simulink model "TempCorrect_OfflineTest"  (R2014a)
settings: Solver=ode3  StartTime=0.0  StopTime=1130  FixedStep=1/400  RelTol=1e-3
settings Model: ExtModeTrigDuration=40001  Creator=darenlee  LastModifiedBy=darenlee
settings DataIOCC: SignalLoggingSaveFormat=ModelDataLogs
settings DebuggingCC: MultiTaskDSMMsg=warning  MultiTaskCondExecSysMsg=none
settings RTWCC: IncludeERTFirstTime=on

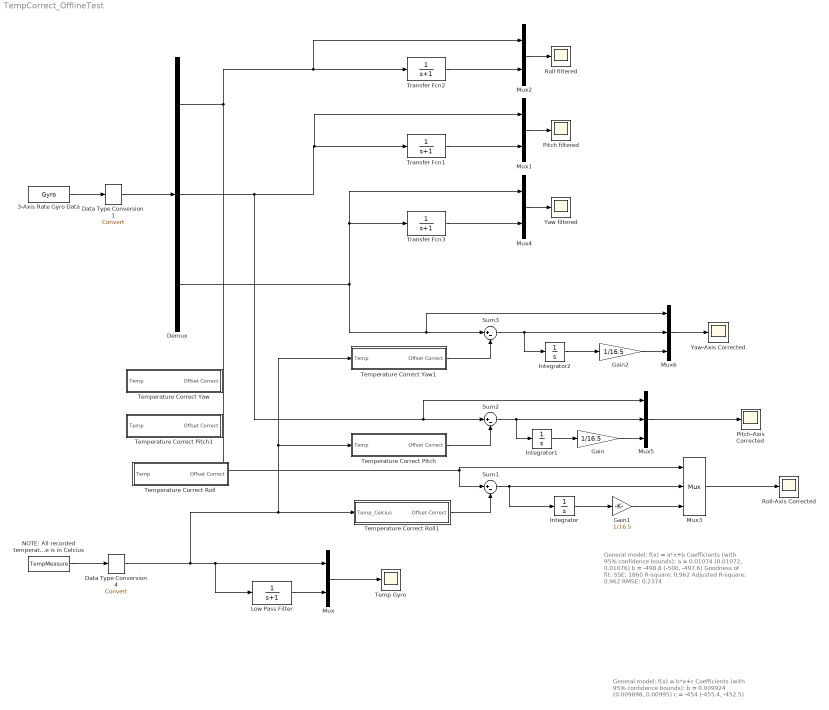
== system TempCorrect_OfflineTest ==
  note: General model:
      |      f(x) = b*x+c
      | Coefficients (with 95% confidence bounds):
      |        b =    0.009924  (0.009898, 0.00995)
      |        c =        -454  (-455.4, -452.5)
  note: General model:
      |      f(x) = a*x+b
      | Coefficients (with 95% confidence bounds):
      |        a =     0.01074  (0.01072, 0.01076)
      |        b =      -498.8  (-500, -497.6)
      |
      | Goodness of fit:
      |   SSE: 1860
      |   R-square: 0.962
      |   Adjusted R-square: 0.962
      |   RMSE: 0.2374
  3-Axis Rate Gyro Data : FromWorkspace  VariableName=Gyro
  Data Type Conversion1 : DataTypeConversion
  Data Type Conversion4 : DataTypeConversion
  Demux : Demux  Outputs=3
  Gain : Gain  Gain=1/16.5
  Gain1 : Gain  Gain=1/16.5
  Gain2 : Gain  Gain=1/16.5
  Integrator : Integrator
  Integrator1 : Integrator
  Integrator2 : Integrator
  Low Pass Filter : TransferFcn  Denominator=[1 1]
  Mux{,1..2,4} (4 alike) : Mux  Inputs=2
  Mux3 : Mux  Inputs=3
  Mux5 : Mux  Inputs=3
  Mux6 : Mux  Inputs=3
  NOTE: All recorded temperature is in Celcius : FromWorkspace  VariableName=TempMeasure
  Pitch filtered : Scope
      settings: SaveName=Pitch_Gyro_filtered
  Pitch-Axis Corrected : Scope
      settings: YMin=-50  YMax=1000  SaveName=Pitch_Corrected_Uncorrected
  Roll filtered : Scope
      settings: SaveName=Roll_Gyro_filtered
  Roll-Axis Corrected : Scope
      settings: TimeRange=571.1351351351351  YMin=-100  YMax=600  SaveName=Roll_Corrected_Uncorrected
  Sum1 : Sum  Inputs=|+-
  Sum2 : Sum  Inputs=|+-
  Sum3 : Sum  Inputs=|+-
  Temp Gyro : Scope
      settings: YMin=0  YMax=55000  SaveName=FilteredTemp
  Temperature Correct Pitch : Subsystem
  Temperature Correct Pitch1 : Subsystem
  Temperature Correct Roll : Subsystem
  Temperature Correct Roll1 : Subsystem
  Temperature Correct Yaw : Subsystem
  Temperature Correct Yaw1 : Subsystem
  Transfer Fcn1 : TransferFcn  Denominator=[1 1]
  Transfer Fcn2 : TransferFcn  Denominator=[1 1]
  Transfer Fcn3 : TransferFcn  Denominator=[1 1]
  Yaw filtered : Scope
      settings: SaveName=Yaw_Gyro_filtered
  Yaw-Axis Corrected : Scope
      settings: YMin=0  YMax=3000  SaveName=Roll_Corrected_Uncorrected2
  wires:
  3-Axis Rate Gyro Data/1 -> Data Type Conversion1/1
  NOTE: All recorded temperature is in Celcius/1 -> Data Type Conversion4/1
  Data Type Conversion1/1 -> Demux/1
  Demux/1 -> Sum1/1, Mux3/1, Mux2/1, Transfer Fcn2/1
  Data Type Conversion4/1 -> Temperature Correct Roll1/1(Temp_Celcius), Temperature Correct Yaw1/1(Temp), Temperature Correct Pitch/1(Temp), Mux/1, Low Pass Filter/1
  Mux/1 -> Temp Gyro/1
  Transfer Fcn2/1 -> Mux2/2
  Sum1/1 -> Integrator/1, Mux3/2
  Mux3/1 -> Roll-Axis Corrected/1
  Mux2/1 -> Roll filtered/1
  Transfer Fcn1/1 -> Mux1/2
  Mux1/1 -> Pitch filtered/1
  Demux/3 -> Mux6/1, Sum3/1, Mux4/1, Transfer Fcn3/1
  Transfer Fcn3/1 -> Mux4/2
  Mux4/1 -> Yaw filtered/1
  Mux5/1 -> Pitch-Axis Corrected/1
  Sum2/1 -> Integrator1/1, Mux5/2
  Low Pass Filter/1 -> Mux/2
  Demux/2 -> Mux5/1, Sum2/1, Mux1/1, Transfer Fcn1/1
  Temperature Correct Pitch/1(Offset Correct) -> Sum2/2
  Temperature Correct Roll1/1(Offset Correct) -> Sum1/2
  Mux6/1 -> Yaw-Axis Corrected/1
  Sum3/1 -> Integrator2/1, Mux6/2
  Temperature Correct Yaw1/1(Offset Correct) -> Sum3/2
  Integrator/1 -> Gain1/1
  Integrator1/1 -> Gain/1
  Gain/1 -> Mux5/3
  Gain1/1 -> Mux3/3
  Integrator2/1 -> Gain2/1
  Gain2/1 -> Mux6/3

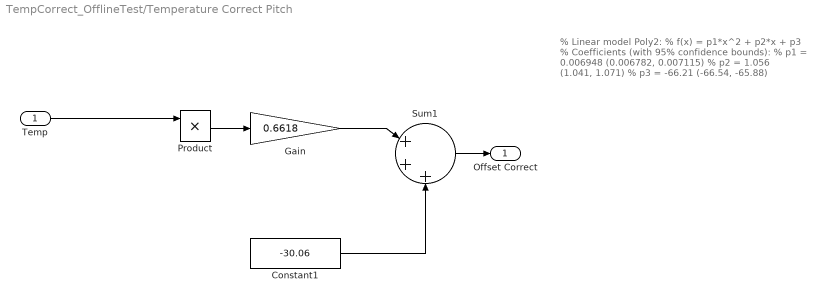
== system TempCorrect_OfflineTest/Temperature Correct Pitch ==
  note: % Linear model Poly2:
      | %      f(x) = p1*x^2 + p2*x + p3
      | % Coefficients (with 95% confidence bounds):
      | %        p1 =    0.006948  (0.006782, 0.007115)
      | %        p2 =       1.056  (1.041, 1.071)
      | %        p3 =      -66.21  (-66.54, -65.88)
  Temp : Inport
  Constant1 : Constant  Value=-30.06
  Gain : Gain  Gain=0.6618
  Product : Product
  Sum1 : Sum  Inputs=|+++
  Offset Correct : Outport
  wires:
  Temp/1 -> Product/1
  Product/1 -> Gain/1
  Gain/1 -> Sum1/1
  Constant1/1 -> Sum1/3
  Sum1/1 -> Offset Correct/1

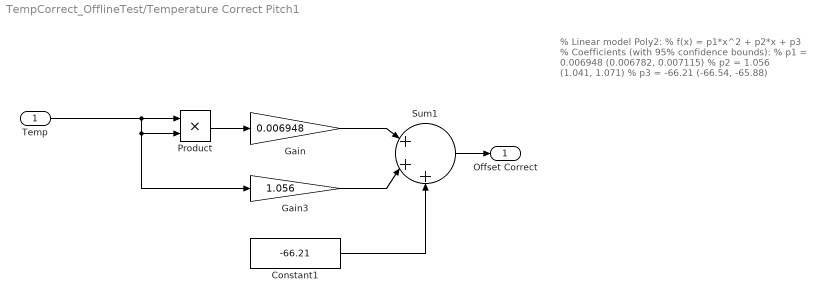
== system TempCorrect_OfflineTest/Temperature Correct Pitch1 ==
  note: % Linear model Poly2:
      | %      f(x) = p1*x^2 + p2*x + p3
      | % Coefficients (with 95% confidence bounds):
      | %        p1 =    0.006948  (0.006782, 0.007115)
      | %        p2 =       1.056  (1.041, 1.071)
      | %        p3 =      -66.21  (-66.54, -65.88)
  Temp : Inport
  Constant1 : Constant  Value=-66.21
  Gain : Gain  Gain=0.006948
  Gain3 : Gain  Gain=1.056
  Product : Product
  Sum1 : Sum  Inputs=|+++
  Offset Correct : Outport
  wires:
  Temp/1 -> Product/1, Gain3/1, Product/2
  Product/1 -> Gain/1
  Gain/1 -> Sum1/1
  Gain3/1 -> Sum1/2
  Constant1/1 -> Sum1/3
  Sum1/1 -> Offset Correct/1

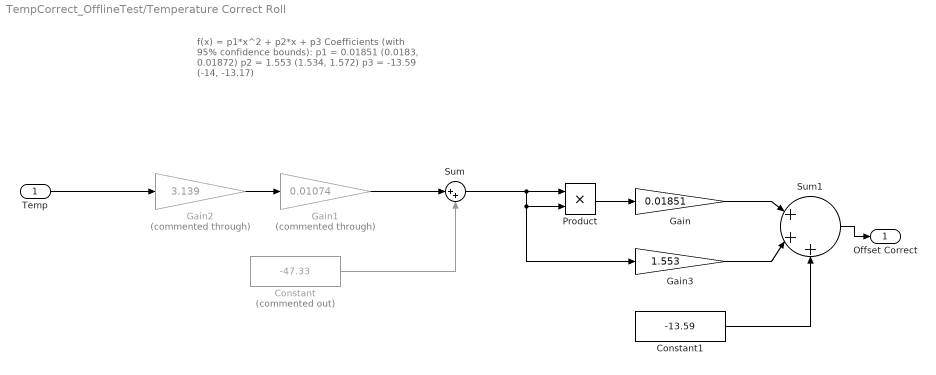
== system TempCorrect_OfflineTest/Temperature Correct Roll ==
  note: f(x) = p1*x^2 + p2*x + p3
      | Coefficients (with 95% confidence bounds):
      |        p1 =     0.01851  (0.0183, 0.01872)
      |        p2 =       1.553  (1.534, 1.572)
      |        p3 =      -13.59  (-14, -13.17)
  Temp : Inport
  Constant : Constant  Commented=on  Value=-47.33
  Constant1 : Constant  Value=-13.59
  Gain : Gain  Gain=0.01851
  Gain1 : Gain  Commented=through  Gain=0.01074
  Gain2 : Gain  Commented=through  Gain=3.139
  Gain3 : Gain  Gain=1.553
  Product : Product
  Sum : Sum  Inputs=|++
  Sum1 : Sum  Inputs=|+++
  Offset Correct : Outport
  wires:
  Gain2/1 -> Gain1/1
  Constant/1 -> Sum/2
  Sum/1 -> Product/1, Gain3/1, Product/2
  Gain1/1 -> Sum/1
  Temp/1 -> Gain2/1
  Product/1 -> Gain/1
  Gain/1 -> Sum1/1
  Gain3/1 -> Sum1/2
  Constant1/1 -> Sum1/3
  Sum1/1 -> Offset Correct/1

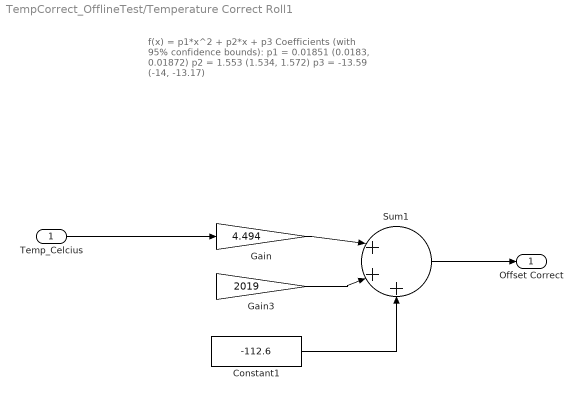
== system TempCorrect_OfflineTest/Temperature Correct Roll1 ==
  note: f(x) = p1*x^2 + p2*x + p3
      | Coefficients (with 95% confidence bounds):
      |        p1 =     0.01851  (0.0183, 0.01872)
      |        p2 =       1.553  (1.534, 1.572)
      |        p3 =      -13.59  (-14, -13.17)
  Temp_Celcius : Inport
  Constant1 : Constant  Value=-112.6
  Gain : Gain  Gain=4.494
  Gain3 : Gain  Gain=2019
  Sum1 : Sum  Inputs=|+++
  Offset Correct : Outport
  wires:
  Temp_Celcius/1 -> Gain/1
  Gain/1 -> Sum1/1
  Gain3/1 -> Sum1/2
  Constant1/1 -> Sum1/3
  Sum1/1 -> Offset Correct/1

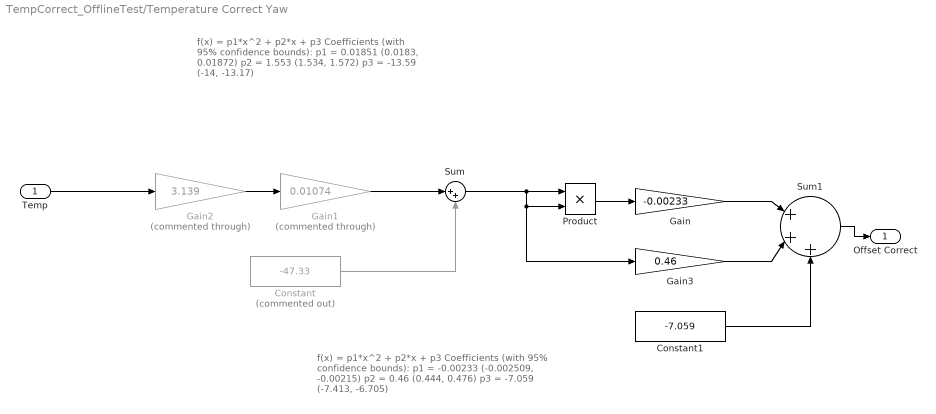
== system TempCorrect_OfflineTest/Temperature Correct Yaw ==
  note: f(x) = p1*x^2 + p2*x + p3
      | Coefficients (with 95% confidence bounds):
      |        p1 =     0.01851  (0.0183, 0.01872)
      |        p2 =       1.553  (1.534, 1.572)
      |        p3 =      -13.59  (-14, -13.17)
  note: f(x) = p1*x^2 + p2*x + p3
      | Coefficients (with 95% confidence bounds):
      |        p1 =    -0.00233  (-0.002509, -0.00215)
      |        p2 =        0.46  (0.444, 0.476)
      |        p3 =      -7.059  (-7.413, -6.705)
  Temp : Inport
  Constant : Constant  Commented=on  Value=-47.33
  Constant1 : Constant  Value=-7.059
  Gain : Gain  Gain=-0.00233
  Gain1 : Gain  Commented=through  Gain=0.01074
  Gain2 : Gain  Commented=through  Gain=3.139
  Gain3 : Gain  Gain=0.46
  Product : Product
  Sum : Sum  Inputs=|++
  Sum1 : Sum  Inputs=|+++
  Offset Correct : Outport
  wires:
  Gain2/1 -> Gain1/1
  Constant/1 -> Sum/2
  Sum/1 -> Product/1, Gain3/1, Product/2
  Gain1/1 -> Sum/1
  Temp/1 -> Gain2/1
  Product/1 -> Gain/1
  Gain/1 -> Sum1/1
  Gain3/1 -> Sum1/2
  Constant1/1 -> Sum1/3
  Sum1/1 -> Offset Correct/1

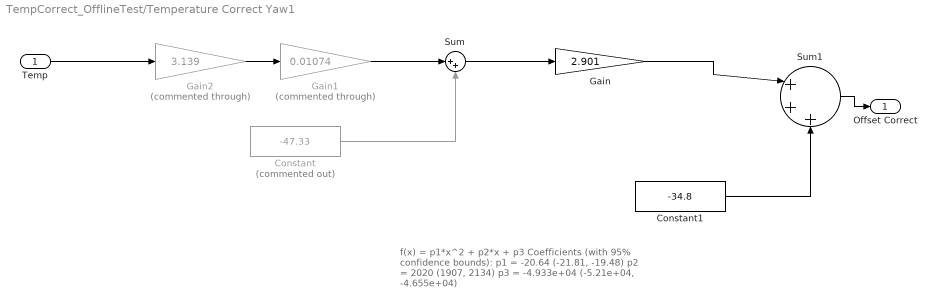
== system TempCorrect_OfflineTest/Temperature Correct Yaw1 ==
  note: f(x) = p1*x^2 + p2*x + p3
      | Coefficients (with 95% confidence bounds):
      |        p1 =      -20.64  (-21.81, -19.48)
      |        p2 =        2020  (1907, 2134)
      |        p3 =  -4.933e+04  (-5.21e+04, -4.655e+04)
  Temp : Inport
  Constant : Constant  Commented=on  Value=-47.33
  Constant1 : Constant  Value=-34.8
  Gain : Gain  Gain=2.901
  Gain1 : Gain  Commented=through  Gain=0.01074
  Gain2 : Gain  Commented=through  Gain=3.139
  Sum : Sum  Inputs=|++
  Sum1 : Sum  Inputs=|+++
  Offset Correct : Outport
  wires:
  Sum1/1 -> Offset Correct/1
  Constant1/1 -> Sum1/3
  Gain/1 -> Sum1/1
  Sum/1 -> Gain/1
  Temp/1 -> Gain2/1
  Gain1/1 -> Sum/1
  Constant/1 -> Sum/2
  Gain2/1 -> Gain1/1
